simulink model "PLC"  (R2025b)
settings: Solver=VariableStepAuto  StartTime=0.0  StopTime=12  RelTol=1e-3

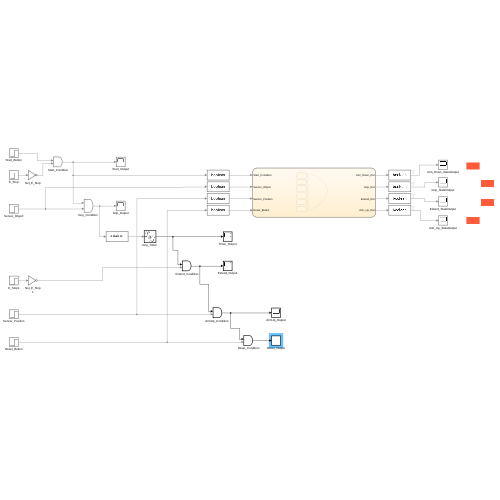
[thumbnail: Simulink's stored preview of the top-level diagram]
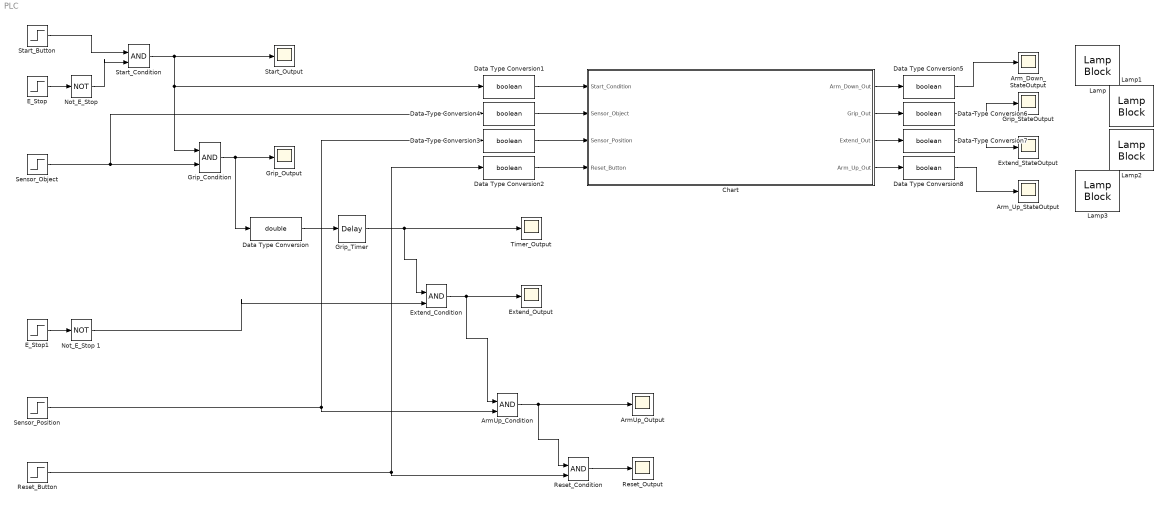
== system PLC ==
  " Extend_Condition" : Logic  IconShape=distinctive  AllPortsSameDT=off  OutDataTypeStr=boolean
  " Reset_Condition" : Logic  IconShape=distinctive  AllPortsSameDT=off  OutDataTypeStr=boolean
  " Start_Condition" : Logic  IconShape=distinctive  AllPortsSameDT=off  OutDataTypeStr=boolean
  "ArmUp_Condition " : Logic  IconShape=distinctive  AllPortsSameDT=off  OutDataTypeStr=boolean
  ArmUp_Output : Scope
      settings: ActiveDisplayYMinimum=-0.12499999999999997  ActiveDisplayYMaximum=1.125  DataLoggingVariableName=ScopeData4
  Arm_Down_StateOutput : Scope
      settings: ActiveDisplayYMinimum=-0.12499999999999997  ActiveDisplayYMaximum=1.125  DataLoggingVariableName=ScopeData6
  Arm_Up_StateOutput : Scope
      settings: ActiveDisplayYMinimum=-0.32764311812788527  ActiveDisplayYMaximum=1.3093162192324295  DataLoggingVariableName=ScopeData7
  Chart : Stateflow chart  TreatAsAtomicUnit=on
  Data Type Conversion : DataTypeConversion  OutDataTypeStr=double  SaturateOnIntegerOverflow=off  RndMeth=Floor
  Data Type Conversion{1..8} (8 alike) : DataTypeConversion  OutDataTypeStr=boolean  SaturateOnIntegerOverflow=off  RndMeth=Floor
  E_Stop : Step  Time=100  SampleTime=0
  E_Stop1 : Step  Time=100  SampleTime=0
  Extend_Output : Scope
      settings: ActiveDisplayYMinimum=-0.12499999999999997  ActiveDisplayYMaximum=1.125  DataLoggingVariableName=ScopeData3
  Extend_StateOutput : Scope
      settings: ActiveDisplayYMinimum=-0.12499999999999997  ActiveDisplayYMaximum=1.125  DataLoggingVariableName=ScopeData8
  "Grip_Condition " : Logic  IconShape=distinctive  AllPortsSameDT=off  OutDataTypeStr=boolean
  Grip_Output : Scope
      settings: ActiveDisplayYMinimum=-0.12499999999999997  ActiveDisplayYMaximum=1.125
  Grip_StateOutput : Scope
      settings: ActiveDisplayYMinimum=-0.12499999999999997  ActiveDisplayYMaximum=1.125  DataLoggingVariableName=ScopeData9
  "Grip_Timer " : TransportDelay  DelayTime=2
  Lamp{,1..3} (4 alike) : LampBlock  LabelPosition=Hide  DefaultColor=[192.0, 192.0, 192.0]  Icon=Rectangle
  "Not_E_Stop " : Logic  Operator=NOT  IconShape=distinctive  AllPortsSameDT=off  OutDataTypeStr=boolean
  Not_E_Stop 1 : Logic  Operator=NOT  IconShape=distinctive  AllPortsSameDT=off  OutDataTypeStr=boolean
  Reset_Button : Step  Time=9  SampleTime=0
  Reset_Output : Scope
      settings: ActiveDisplayYMinimum=-0.12499999999999997  ActiveDisplayYMaximum=1.125  DataLoggingVariableName=ScopeData5
  Sensor_Object : Step  Time=3  SampleTime=0
  Sensor_Position : Step  Time=7  SampleTime=0
  Start_Button : Step  SampleTime=0
  Start_Output : Scope
      settings: ActiveDisplayYMinimum=-0.12499999999999997  ActiveDisplayYMaximum=1.125
  Timer_Output : Scope
      settings: ActiveDisplayYMinimum=-0.12499999999999997  ActiveDisplayYMaximum=1.125  DataLoggingVariableName=ScopeData2
  wires:
  E_Stop/1 -> "Not_E_Stop "/1
  "Not_E_Stop "/1 -> " Start_Condition"/2
  Start_Button/1 -> " Start_Condition"/1
  "Grip_Condition "/1 -> Data Type Conversion/1, Grip_Output/1
  " Start_Condition"/1 -> Data Type Conversion1/1, "Grip_Condition "/1, Start_Output/1
  "Grip_Timer "/1 -> " Extend_Condition"/1, Timer_Output/1
  Data Type Conversion/1 -> "Grip_Timer "/1
  E_Stop1/1 -> Not_E_Stop 1/1
  Not_E_Stop 1/1 -> " Extend_Condition"/2
  " Extend_Condition"/1 -> "ArmUp_Condition "/1, Extend_Output/1
  Sensor_Position/1 -> "ArmUp_Condition "/2, Data Type Conversion3/1
  "ArmUp_Condition "/1 -> " Reset_Condition"/1, ArmUp_Output/1
  Reset_Button/1 -> " Reset_Condition"/2, Data Type Conversion2/1
  " Reset_Condition"/1 -> Reset_Output/1
  Sensor_Object/1 -> Data Type Conversion4/1, "Grip_Condition "/2
  Chart/1(Arm_Down_Out) -> Data Type Conversion5/1
  Chart/2(Grip_Out) -> Data Type Conversion6/1
  Chart/3(Extend_Out) -> Data Type Conversion7/1
  Chart/4(Arm_Up_Out) -> Data Type Conversion8/1
  Data Type Conversion1/1 -> Chart/1(Start_Condition)
  Data Type Conversion4/1 -> Chart/2(Sensor_Object)
  Data Type Conversion3/1 -> Chart/3(Sensor_Position)
  Data Type Conversion2/1 -> Chart/4(Reset_Button)
  Data Type Conversion8/1 -> Arm_Up_StateOutput/1
  Data Type Conversion7/1 -> Extend_StateOutput/1
  Data Type Conversion6/1 -> Grip_StateOutput/1
  Data Type Conversion5/1 -> Arm_Down_StateOutput/1

== stateflow chart PLC/Chart ==
  state Idle
    entry:
    Arm_Down_Out = false;
    Grip_Out = false;
    Extend_Out = false;
    Arm_Up_Out = false;
  state Arm_Down
    entry:
    Arm_Down_Out = true;
    Grip_Out = false;
    Extend_Out = false;
    Arm_Up_Out = false;
  state Grip
    entry:
    Arm_Down_Out = false;
    Grip_Out = true;
    Extend_Out = false;
    Arm_Up_Out = false;
  state Extend
    entry:
    Arm_Down_Out = false;
    Grip_Out = false;
    Extend_Out = true;
    Arm_Up_Out = false;
  state Arm_Up
    entry:
    Arm_Down_Out = false;
    Grip_Out = false;
    Extend_Out = false;
    Arm_Up_Out = true;
  state Reset
    entry:
    Arm_Down_Out = false;
    Grip_Out = false;
    Extend_Out = false;
    Arm_Up_Out = false;
  Reset -> Idle : [Reset_Button == 1]
  Idle -> Arm_Down : [Start_Condition == 1]
  (default) -> Idle
  Arm_Down -> Grip : [Sensor_Object == 1]
  Grip -> Extend : [after(4, sec)]
  Extend -> Arm_Up : [after(2, sec)]
  Arm_Up -> Reset : [after(3, sec)]
  data: Start_Condition input boolean; Sensor_Object input boolean; Sensor_Position input boolean; Reset_Button input boolean; Arm_Down_Out output boolean; Grip_Out output boolean; Extend_Out output boolean; Arm_Up_Out output boolean
